simulink model "tut04c"  (R2024b)
settings: Solver=VariableStepAuto  StartTime=0.0  StopTime=10.0  RelTol=1e-3
libraries: NSA_DEVS_LOGISTICS_ATOMIC x8, NSA_DEVS_SINKS_ATOMIC x6, NSA_DEVS_STATISTICS_ATOMIC x1, NSA_DEVS_MATH_OPERATIONS_ATOMIC x1, NSA_DEVS_ROUTING_ATOMIC x1, NSA_DEVS_SOURCES_ATOMIC x1
settings Model: Creator=peter  LastModifiedBy=peter

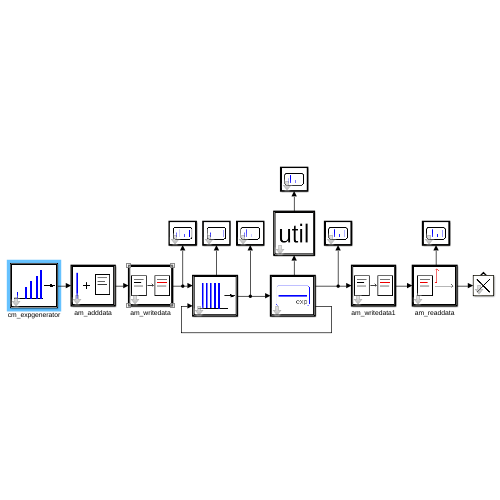
[thumbnail: Simulink's stored preview of the top-level diagram]
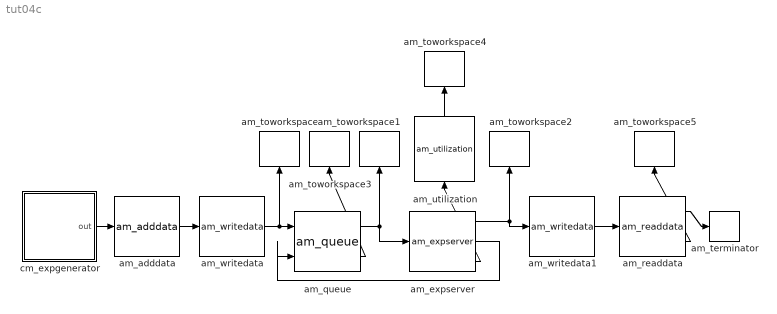
== system tut04c ==
  am_adddata : NSA_DEVS_LOGISTICS_ATOMIC/am_adddata  fields="[\"startTime\"]"  values=[0]  numeric=[true]  infield="\"id\""  tau=[0,1]  debug=0
      settings: SourceProductName=Atomic
  am_expserver : NSA_DEVS_LOGISTICS_ATOMIC/am_expserver  tS=0.9  useSeed=false  seed=0  tau=[0,1]  debug=0
      settings: SourceProductName=Atomic
  am_queue : NSA_DEVS_LOGISTICS_ATOMIC/am_queue  tD=[0,2]  tau=[0,1]  debug=0
      settings: SourceProductName=Atomic
  am_readdata : NSA_DEVS_LOGISTICS_ATOMIC/am_readdata  field="\"startTime\""  tau=[0,1]  debug=0
      settings: SourceProductName=Atomic
  am_terminator : NSA_DEVS_LOGISTICS_ATOMIC/am_terminator  tau=[0,1]  debug=0
      settings: SourceProductName=Atomic
  am_toworkspace : NSA_DEVS_SINKS_ATOMIC/am_toworkspace  varname="\"gen\""  t0=0  format="\"vector\""  tau=[0,5]  debug=0
      settings: SourceProductName=Atomic
  am_toworkspace1 : NSA_DEVS_SINKS_ATOMIC/am_toworkspace  varname="\"srvIn\""  t0=0  format="\"vector\""  tau=[0,5]  debug=0
      settings: SourceProductName=Atomic
  am_toworkspace2 : NSA_DEVS_SINKS_ATOMIC/am_toworkspace  varname="\"srvOut\""  t0=0  format="\"vector\""  tau=[0,5]  debug=0
      settings: SourceProductName=Atomic
  am_toworkspace3 : NSA_DEVS_SINKS_ATOMIC/am_toworkspace  varname="\"qLen\""  t0=0  format="\"vector\""  tau=[0,5]  debug=0
      settings: SourceProductName=Atomic
  am_toworkspace4 : NSA_DEVS_SINKS_ATOMIC/am_toworkspace  varname="\"sUtil\""  t0=0  format="\"vector\""  tau=[0,5]  debug=0
      settings: SourceProductName=Atomic
  am_toworkspace5 : NSA_DEVS_SINKS_ATOMIC/am_toworkspace  varname="\"eTime\""  t0=0  format="\"vector\""  tau=[0,5]  debug=0
      settings: SourceProductName=Atomic
  am_utilization : NSA_DEVS_STATISTICS_ATOMIC/am_utilization  tau=[0,1]  debug=0
      settings: SourceProductName=Atomic
  am_writedata : NSA_DEVS_LOGISTICS_ATOMIC/am_writedata  inFields=[]  outField="\"startTime\""  changeFunc="\"out = get_time();\""  tau=[0,1]  debug=0
      settings: SourceProductName=Atomic
  am_writedata1 : NSA_DEVS_LOGISTICS_ATOMIC/am_writedata  inFields="\"startTime\""  outField="\"startTime\""  changeFunc="\"out = get_time() - in(1);\""  tau=[0,1]  debug=0
      settings: SourceProductName=Atomic
  cm_expgenerator : Subsystem  mask(ExpGenerator){tS=1.1, useSeed=false, seed=0}
      mask prompts: tS "mean service time"; useSeed "use seed"
      mask help: Generates entities with exponentially distributed interarrival times and increasing id's.
      mask Help:
      | <p>Generates entities with exponentially distributed interarrival times and increasing id's.</p>
      | 
      | <p>Ports
      | <ul>
      | <li>outputs:
      |   <ul>
      |     <li>out: outgoing entities</li>
      |   </ul>
      | </li>
      | </ul>
      | </p>
      | 
      | <p>Parameters
      | <ul>
      | <li>tS:  mean service time</li>
      | <li>useSeed:  true -> seed is used in constructor</li>
      | <li>seed: seed of random generator</li>
      | </ul>
      | </p>
      mask Display: image('icon_expgenerator.png');
  wires:
  am_expserver/1 -> am_writedata1/1, am_toworkspace2/1
  am_expserver/2 -> am_queue/2
  am_queue/1 -> am_toworkspace1/1, am_expserver/1
  am_queue/2 -> am_toworkspace3/1
  am_utilization/1 -> am_toworkspace4/1
  am_expserver/3 -> am_utilization/1
  am_adddata/1 -> am_writedata/1
  am_writedata/1 -> am_queue/1, am_toworkspace/1
  am_writedata1/1 -> am_readdata/1
  am_readdata/1 -> am_terminator/1
  am_readdata/2 -> am_toworkspace5/1
  cm_expgenerator/1(out) -> am_adddata/1

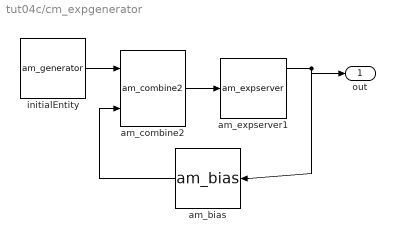
== system tut04c/cm_expgenerator ==
  am_bias : NSA_DEVS_MATH_OPERATIONS_ATOMIC/am_bias  bias=1  tau=[0,1]  debug=0
      settings: SourceProductName=Atomic
  am_combine2 : NSA_DEVS_ROUTING_ATOMIC/am_combine2  tD=[0,2]  tau=[0,1]  debug=0
      settings: SourceProductName=Atomic
  am_expserver1 : NSA_DEVS_LOGISTICS_ATOMIC/am_expserver  tS=tS  useSeed=useSeed  seed=seed  tau=[0,1]  debug=0
      settings: SourceProductName=Atomic
  initialEntity : NSA_DEVS_SOURCES_ATOMIC/am_generator  tG=0  n0=1  nG=1  tD=[0,2]  debug=0
      settings: SourceProductName=Atomic
  out : Outport
  wires:
  am_bias/1 -> am_combine2/2
  initialEntity/1 -> am_combine2/1
  am_combine2/1 -> am_expserver1/1
  am_expserver1/1 -> out/1, am_bias/1
